simulink model "NOLCO2"  (R2017b)
settings: Solver=VariableStepAuto  StartTime=0.0  StopTime=20.0  FixedStep=0.001  RelTol=1e-3
values from neighbouring files (symbols this model uses):
  Kx = -[1000 4000 600 40]    [config2.m]
  Kz = Kx    [config2.m]
settings Model: Creator=lbergantin2017  LastModifiedBy=miche
settings CodeAppCC: StateflowObjectComments=on

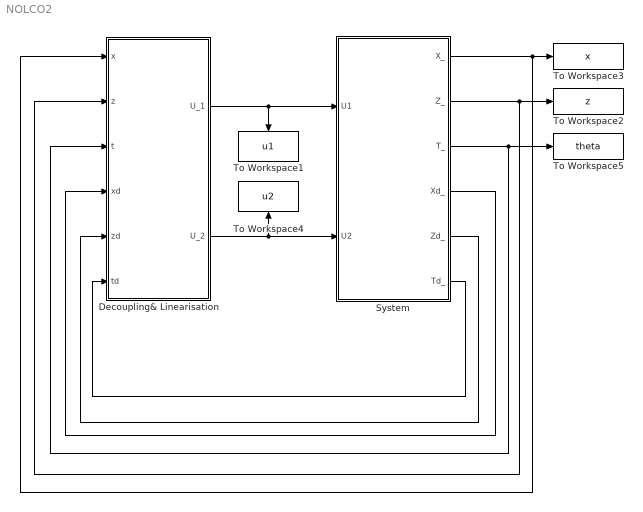
== system NOLCO2 ==
  Decoupling& Linearisation : Subsystem
  System : Subsystem
  To Workspace1 : ToWorkspace  VariableName=u1  SampleTime=-1
  To Workspace2 : ToWorkspace  VariableName=z  SampleTime=-1
  To Workspace3 : ToWorkspace  VariableName=x  SampleTime=-1
  To Workspace4 : ToWorkspace  VariableName=u2  SampleTime=-1
  To Workspace5 : ToWorkspace  VariableName=theta  SampleTime=-1
  wires:
  Decoupling& Linearisation/1(U_1) -> To Workspace1/1, System/1("U1 ")
  System/1(X_) -> To Workspace3/1, Decoupling& Linearisation/1(x)
  System/2("Z_ ") -> Decoupling& Linearisation/2(z), To Workspace2/1
  Decoupling& Linearisation/2(U_2) -> System/2(U2), To Workspace4/1
  System/3(T_) -> Decoupling& Linearisation/3("t "), To Workspace5/1
  System/4(Xd_) -> Decoupling& Linearisation/4(xd)
  System/5(Zd_) -> Decoupling& Linearisation/5(zd)
  System/6(Td_) -> Decoupling& Linearisation/6(td)

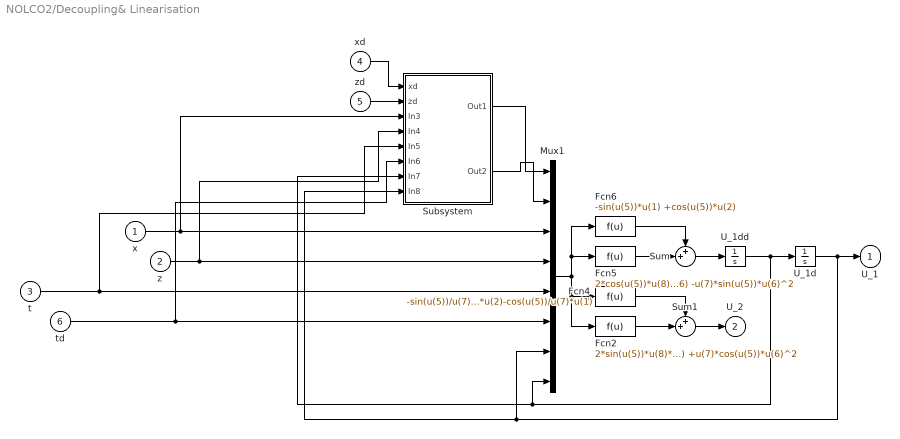
== system NOLCO2/Decoupling& Linearisation ==
  x : Inport
  z : Inport  Port=2
  "t " : Inport  Port=3
  xd : Inport  Port=4
  zd : Inport  Port=5
  td : Inport  Port=6
  Fcn2 : Fcn  Expr=2*sin(u(5))*u(8)*u(6) +u(7)*cos(u(5))*u(6)^2
  Fcn4 : Fcn  Expr=-sin(u(5))/u(7)*u(2)-cos(u(5))/u(7)*u(1)
  Fcn5 : Fcn  Expr=2*cos(u(5))*u(8)*u(6) -u(7)*sin(u(5))*u(6)^2
  Fcn6 : Fcn  Expr=-sin(u(5))*u(1) +cos(u(5))*u(2)
  Mux1 : Mux  Inputs=8
  Subsystem : Subsystem
  Sum : Sum  Inputs=++|
  Sum1 : Sum  Inputs=++|
  U_1d : Integrator  InitialCondition=1
  U_1dd : Integrator
  U_1 : Outport
  U_2 : Outport  Port=2
  wires:
  x/1 -> Subsystem/3(In3), Mux1/3
  "t "/1 -> Subsystem/5(In5), Mux1/5
  Mux1/1 -> Fcn2/1, Fcn4/1, Fcn5/1, Fcn6/1
  z/1 -> Subsystem/4(In4), Mux1/4
  Fcn6/1 -> Sum/1
  Fcn5/1 -> Sum/2
  td/1 -> Subsystem/6(In6), Mux1/6
  Sum/1 -> U_1dd/1
  U_1dd/1 -> Subsystem/7(In7), Mux1/8, U_1d/1
  U_1d/1 -> Subsystem/8(In8), Mux1/7, U_1/1
  Sum1/1 -> U_2/1
  Fcn2/1 -> Sum1/2
  Fcn4/1 -> Sum1/1
  xd/1 -> Subsystem/1(xd)
  zd/1 -> Subsystem/2(zd)
  Subsystem/1(Out1) -> Mux1/1
  Subsystem/2(Out2) -> Mux1/2

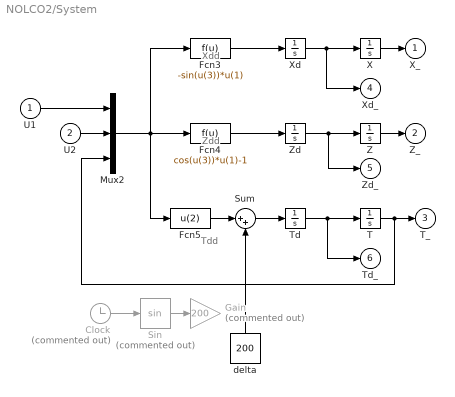
== system NOLCO2/System ==
  note: Xdd
  note: Zdd
  note: Tdd
  "U1 " : Inport
  U2 : Inport  Port=2
  Clock : Clock  Commented=on
  Fcn3 : Fcn  Expr=-sin(u(3))*u(1)
  Fcn4 : Fcn  Expr=cos(u(3))*u(1)-1
  Fcn5 : Fcn  Expr=u(2)
  Gain : Gain  Commented=on  Gain=200
  Mux2 : Mux  Inputs=3
  Sin : Trigonometry  Commented=on
  Sum : Sum  Inputs=|++
  T : Integrator  InitialCondition=1
  Td : Integrator  InitialCondition=1
  X : Integrator  InitialCondition=1
  Xd : Integrator
  Z : Integrator  InitialCondition=1
  Zd : Integrator
  delta : Constant  Value=200
  X_ : Outport
  "Z_ " : Outport  Port=2
  T_ : Outport  Port=3
  Xd_ : Outport  Port=4
  Zd_ : Outport  Port=5
  Td_ : Outport  Port=6
  wires:
  Fcn3/1 -> Xd/1
  Xd/1 -> Xd_/1, X/1
  Zd/1 -> Zd_/1, Z/1
  Fcn4/1 -> Zd/1
  Mux2/1 -> Fcn5/1, Fcn3/1, Fcn4/1
  Td/1 -> Td_/1, T/1
  "U1 "/1 -> Mux2/1
  U2/1 -> Mux2/2
  X/1 -> X_/1
  Z/1 -> "Z_ "/1
  T/1 -> T_/1, Mux2/3
  Sum/1 -> Td/1
  Fcn5/1 -> Sum/1
  Clock/1 -> Sin/1
  Sin/1 -> Gain/1
  delta/1 -> Sum/2

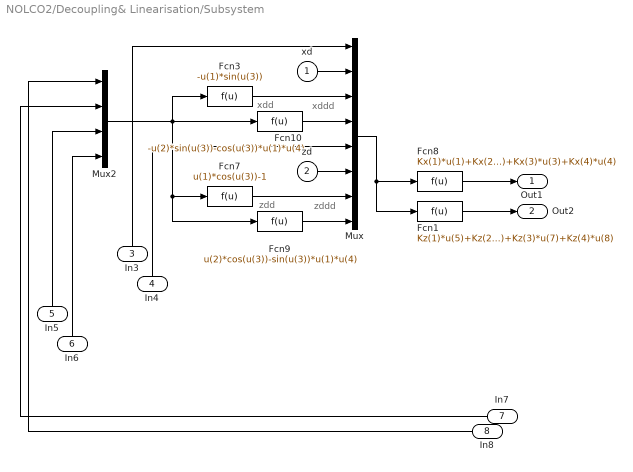
== system NOLCO2/Decoupling& Linearisation/Subsystem ==
  note: zddd
  note: xddd
  note: xdd
  note: zdd
  xd : Inport
  zd : Inport  Port=2
  In3 : Inport  Port=3
  In4 : Inport  Port=4
  In5 : Inport  Port=5
  In6 : Inport  Port=6
  In7 : Inport  Port=7
  In8 : Inport  Port=8
  Fcn1 : Fcn  Expr=Kz(1)*u(5)+Kz(2)*u(6)+Kz(3)*u(7)+Kz(4)*u(8)
  Fcn10 : Fcn  Expr=-u(2)*sin(u(3))-cos(u(3))*u(1)*u(4)
  Fcn3 : Fcn  Expr=-u(1)*sin(u(3))
  Fcn7 : Fcn  Expr=u(1)*cos(u(3))-1
  Fcn8 : Fcn  Expr=Kx(1)*u(1)+Kx(2)*u(2)+Kx(3)*u(3)+Kx(4)*u(4)
  Fcn9 : Fcn  Expr=u(2)*cos(u(3))-sin(u(3))*u(1)*u(4)
  Mux : Mux  Inputs=8
  Mux2 : Mux
  Out1 : Outport
  Out2 : Outport  Port=2
  wires:
  xd/1 -> Mux/2
  Fcn8/1 -> Out1/1
  In8/1 -> Mux2/1
  In3/1 -> Mux/1
  Fcn3/1 -> Mux/3
  Fcn7/1 -> Mux/7
  zd/1 -> Mux/6
  Mux/1 -> Fcn1/1, Fcn8/1
  In5/1 -> Mux2/3
  In7/1 -> Mux2/2
  In6/1 -> Mux2/4
  In4/1 -> Mux/5
  Mux2/1 -> Fcn3/1, Fcn7/1, Fcn9/1, Fcn10/1
  Fcn1/1 -> Out2/1
  Fcn10/1 -> Mux/4
  Fcn9/1 -> Mux/8
